simulink model "psb2machinesSVC_PSS"  (Simulink 6.0)
settings: Solver=ode23tb  StartTime=0.0  StopTime=10  MaxStep=1/60  RelTol=1e-3
InitFcn:
  | powericon('psbinitsys',bdroot);
undefined symbols (not defined in the file or in its folder): D1, Delta, gcbh, powericon
libraries: powerlib2 x23, powerlib_extras x5
settings Model: Creator=sybille  LastModifiedBy=batserve  ExtModeTrigMode=oneshot  ExtModeArmWhenConnect=off  ExtModeAutoUpdateStatusClock=off
settings DataIOCC: LimitDataPoints=off  SignalLoggingName=sigsOut
settings OptimizationCC: BlockReduction=off  BooleanDataType=off
settings DebuggingCC: SolverPrmCheckMsg=none
settings HardwareCC: TargetUnknown=on

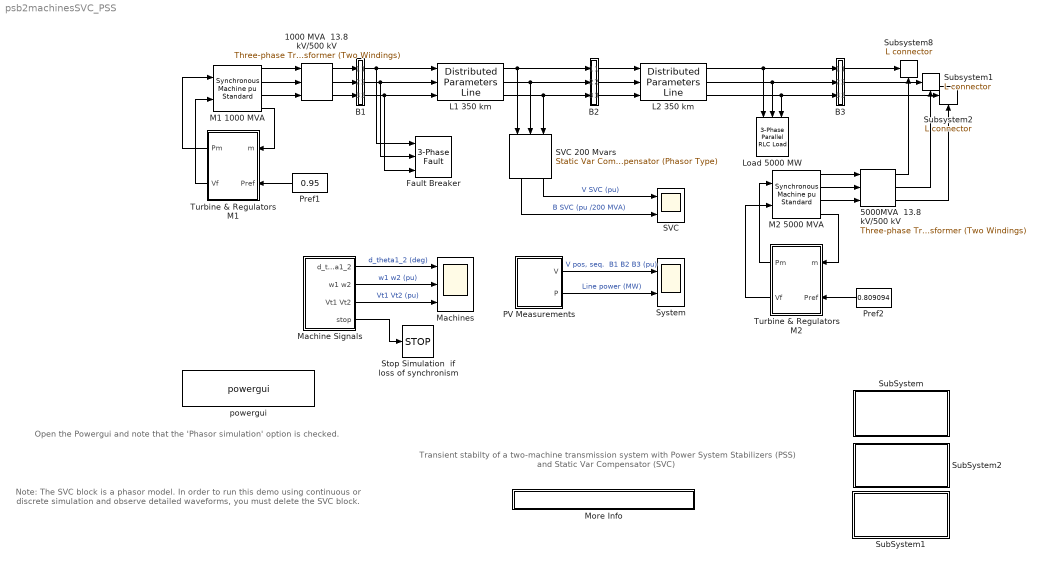
== system psb2machinesSVC_PSS ==
  note: Transient stabilty of a two-machine transmission system
      | with Power System Stabilizers (PSS)
      | and Static Var Compensator (SVC)
  note: Open the Powergui and note
      | that the 'Phasor simulation'
      | option is checked.
  note: Note:
      | The SVC block is a phasor model.
      | In order to run this demo using
      | continuous or discrete simulation
      | and observe detailed waveforms,
      | you must delete the SVC block.
  1000 MVA  13.8 kV/500 kV : powerlib2/Elements/Three-phase Transformer (Two Windings)  Tag=PoWeRsYsTeMbLoCk  nominal=[ 1000e6 60 ]  type1=Delta (D1)  params1="[ 13.8e3 0.002  0.0]"  type2=Yg  params2=[ 500e3 0.002 0.12]  ynsat=off  rmag=500  lm=500  sat="[ 0,0  ;  0.005,1.2  ;  1.0,1.4 ]"  hyst=off  matfile='hysteresis'  sif=off  phi0=[ 0.8 , -0.8 , 0.7 ]  initialslopes=[+1 +1 +1]  mesure=None  PSBOutputType=1111
  5000MVA  13.8 kV/500 kV : powerlib2/Elements/Three-phase Transformer (Two Windings)  Tag=PoWeRsYsTeMbLoCk  nominal=[ 5000e6 60 ]  type1=Delta (D1)  params1="[ 13.8e3 0.002  0.0]"  type2=Yg  params2=[ 500e3 0.002 0.12]  ynsat=off  rmag=500  lm=500  sat="[ 0,0  ;  0.005,1.2  ;  1.0,1.4 ]"  hyst=off  matfile='hysteresis'  sif=off  phi0=[ 0.8 , -0.8 , 0.7 ]  initialslopes=[+1 +1 +1]  mesure=None  PSBOutputType=1111
  B1 : Subsystem  Tag=PoWeRsYsTeMmEaSuReMeNt  AncestorBlock=powerlib2/Measurements/Three-Phase V-I Measurement  LoadFcn=powericon('psbloadfunction',gcbh,'3-Phase VI Measurement','');  InitFcn=powericon('checksum',bdroot)  mask(3-Phase VI Measurement){VChoice=phase-to-ground, ualv=on, labelV=Vabc_B1, Vpu=on, Vbase=500e3, IChoice=yes, ualc=on, labelC=Iabc_B1, Ppu=on, Pbase=100e6, OutputType=Complex, PhasorSimulation=on, PSBequivalent=0, PSBOutputType=11100}
      mask prompts: VChoice "Voltage measurement"; ualv "Use a label"; labelV "Signal label  (use a From block to collect signal)"; Vpu "Voltage  in pu"; Vbase "Base voltage (Vrms phase-phase) :"; IChoice "Current measurement"; ualc "Use a label"; labelC "Signal label  (use a From block to collect signal)"; Ppu "Currents in pu"; Pbase "Base power ( VA 3 phase)"; OutputType "Output signal :"; PhasorSimulation "Phasor simulation"; PSBequivalent "Equivalent circuit"
      mask help:
      | This block is used to measure three-phase voltages and currents in a circuit. When connected in series with a three-phase element, it return the three phase-to-ground voltages and line currents.
      |
      | The block can output the voltages and currents in per unit values or in volts and amperes. Check the appropriate boxes if you want to output the voltages and currents  in pu
      mask init:
      | powericon('psbcallbacks',gcb,'Three-phase measurements',4);
      | if  Vpu
      |     xKv=1/(Vbase/sqrt(3)*sqrt(2));
      | else
      |     xKv=1;
      | end
      | if  Ppu
      |     xKi=1/(Pbase/Vbase/sqrt(3)*sqrt(2));
      | else
      |     xKi=1;
      | end
      | switch OutputType
      | case 1
      |     OutputSelection  = [1:6];
      |     PhasorModeV = [1:3];
      |     NormalModeV = [7:9];
      |     PhasorModeI = [4:6];
      |     NormalModeI = [10:12];
      |     Kv = xKv;
      |     Ki = xKi;
      | case 2
      |     OutputSelection = [7,13,8,14,9,15,10,16,11,17,12,18];
      |     PhasorModeV = [1:6];
      |     NormalModeV = [13:15];
      |     PhasorModeI = [7:12];
      |     NormalModeI = [16:18];
      |     Kv = xKv;
      |     Ki = xKi;
      | case 3
      |     OutputSelection = [13,19,14,20,15,21,16,22,17,23,18,24];
      |     PhasorModeV = [1:6];
      |     NormalModeV = [13:15];
      |     PhasorModeI = [7:12];
      |     NormalModeI = [16:18];
      |     Kv = [xKv 1 xKv 1 xKv 1];
      |     Ki = [xKi 1 xKi 1 xKi 1];
      | case 4
      |     OutputSelection  = [19:24];
      |     PhasorModeV = [1:3];
      |     NormalModeV = [7:9];
      |     PhasorModeI = [4:6];
      |     NormalModeI = [10:12];
      |     Kv = xKv;
      |     Ki = xKi;
      | end
      | if PhasorSimulation
      |     SelectionModeV = PhasorModeV;
      |     SelectionModeI = PhasorModeI;
      | else
      |     SelectionModeV = NormalModeV;
      |     SelectionModeI = NormalModeI;
      |     Kv = xKv;
      |     Ki = xKi;
      | end
      settings: CopyFcn=powericon('psbloadfunction',gcbh,'3-Phase VI Measurement','VerifyPhasor');  CloseFcn=%3phaseVImeasurement
      mask Help: web(psbhelp)
      mask StyleString: popup(no|phase-to-ground|phase-to-phase),checkbox,edit,checkbox,edit,popup(no|yes),checkbox,edit,checkbox,edit,popup(Complex|Real-Imag|Magnitude-Angle|Magnitude),checkbox,edit,edit
      mask CallbackString: powericon('psbcallbacks',gcb,'Three-phase measurements',2);|powericon('psbcallbacks',gcb,'Three-phase measurements',2);||powericon('psbcallbacks',gcb,'Three-phase measurements',2);||powericon('psbcallbacks',gcb,'Three-phase measurements',2);|powericon('psbcallbacks',gcb,'Three-phase measurements',2);||powericon('psbcallbacks',gcb,'Three-phase measurements',4);|||||
  B2 : Subsystem  Tag=PoWeRsYsTeMmEaSuReMeNt  AncestorBlock=powerlib2/Measurements/Three-Phase V-I Measurement  LoadFcn=powericon('psbloadfunction',gcbh,'3-Phase VI Measurement','');  InitFcn=powericon('checksum',bdroot)  mask(3-Phase VI Measurement){VChoice=phase-to-ground, ualv=on, labelV=Vabc_B2, Vpu=on, Vbase=500e3, IChoice=no, ualc=off, labelC=I1, Ppu=off, Pbase=100e6, OutputType=Complex, PhasorSimulation=on, PSBequivalent=0, PSBOutputType=11100}
      mask prompts: VChoice "Voltage measurement"; ualv "Use a label"; labelV "Signal label  (use a From block to collect signal)"; Vpu "Voltage  in pu"; Vbase "Base voltage (Vrms phase-phase) :"; IChoice "Current measurement"; ualc "Use a label"; labelC "Signal label  (use a From block to collect signal)"; Ppu "Currents in pu"; Pbase "Base power ( VA 3 phase)"; OutputType "Output signal :"; PhasorSimulation "Phasor simulation"; PSBequivalent "Equivalent circuit"
      mask help:
      | This block is used to measure three-phase voltages and currents in a circuit. When connected in series with a three-phase element, it return the three phase-to-ground voltages and line currents.
      |
      | The block can output the voltages and currents in per unit values or in volts and amperes. Check the appropriate boxes if you want to output the voltages and currents  in pu
      mask init: same as psb2machinesSVC_PSS/B1
      settings: CopyFcn=powericon('psbloadfunction',gcbh,'3-Phase VI Measurement','VerifyPhasor');  CloseFcn=%3phaseVImeasurement
      mask Help: web(psbhelp)
      mask StyleString: popup(no|phase-to-ground|phase-to-phase),checkbox,edit,checkbox,edit,popup(no|yes),checkbox,edit,checkbox,edit,popup(Complex|Real-Imag|Magnitude-Angle|Magnitude),checkbox,edit,edit
      mask CallbackString: powericon('psbcallbacks',gcb,'Three-phase measurements',2);|powericon('psbcallbacks',gcb,'Three-phase measurements',2);||powericon('psbcallbacks',gcb,'Three-phase measurements',2);||powericon('psbcallbacks',gcb,'Three-phase measurements',2);|powericon('psbcallbacks',gcb,'Three-phase measurements',2);||powericon('psbcallbacks',gcb,'Three-phase measurements',4);|||||
  B3 : Subsystem  Tag=PoWeRsYsTeMmEaSuReMeNt  AncestorBlock=powerlib2/Measurements/Three-Phase V-I Measurement  LoadFcn=powericon('psbloadfunction',gcbh,'3-Phase VI Measurement','');  InitFcn=powericon('checksum',bdroot)  mask(3-Phase VI Measurement){VChoice=phase-to-ground, ualv=on, labelV=Vabc_B3, Vpu=on, Vbase=500e3, IChoice=no, ualc=off, labelC=I1, Ppu=off, Pbase=100e6, OutputType=Complex, PhasorSimulation=on, PSBequivalent=0, PSBOutputType=11100}
      mask prompts: VChoice "Voltage measurement"; ualv "Use a label"; labelV "Signal label  (use a From block to collect signal)"; Vpu "Voltage  in pu"; Vbase "Base voltage (Vrms phase-phase) :"; IChoice "Current measurement"; ualc "Use a label"; labelC "Signal label  (use a From block to collect signal)"; Ppu "Currents in pu"; Pbase "Base power ( VA 3 phase)"; OutputType "Output signal :"; PhasorSimulation "Phasor simulation"; PSBequivalent "Equivalent circuit"
      mask help:
      | This block is used to measure three-phase voltages and currents in a circuit. When connected in series with a three-phase element, it return the three phase-to-ground voltages and line currents.
      |
      | The block can output the voltages and currents in per unit values or in volts and amperes. Check the appropriate boxes if you want to output the voltages and currents  in pu
      mask init: same as psb2machinesSVC_PSS/B1
      settings: CopyFcn=powericon('psbloadfunction',gcbh,'3-Phase VI Measurement','VerifyPhasor');  CloseFcn=%3phaseVImeasurement
      mask Help: web(psbhelp)
      mask StyleString: popup(no|phase-to-ground|phase-to-phase),checkbox,edit,checkbox,edit,popup(no|yes),checkbox,edit,checkbox,edit,popup(Complex|Real-Imag|Magnitude-Angle|Magnitude),checkbox,edit,edit
      mask CallbackString: powericon('psbcallbacks',gcb,'Three-phase measurements',2);|powericon('psbcallbacks',gcb,'Three-phase measurements',2);||powericon('psbcallbacks',gcb,'Three-phase measurements',2);||powericon('psbcallbacks',gcb,'Three-phase measurements',2);|powericon('psbcallbacks',gcb,'Three-phase measurements',2);||powericon('psbcallbacks',gcb,'Three-phase measurements',4);|||||
  Fault Breaker : powerlib2/Elements/3-Phase Fault  sa=on  sb=off  sc=off  Rdef=0.001  st=on  Rt=0.001  comext=off  sw_status=[1 0]  sw_times=[ 0.1 0.1+6.0/60]  Ts=0  init_statext=[0 0 1]  Rp=1e6  Cp=inf  mesure=None
  L1 350 km : powerlib2/Elements/Distributed Parameters Line  Tag=PoWeRsYsTeMbLoCk  n=3  f=60  r="[0.01755  0.2758]"  l="[0.8737e-3  3.220e-3]"  c="[13.33e-9  8.297e-9]"  lgt=350  x1=[0 -1.745e-008 4.874e+005 -1.124e+005;0.0003618 -1.101e-008 4.982e+005 -4.51e+004;0.0007236 -4.365e-009 4.997e+005 2.307e+004;0.001085 2.363e-009 4.919e+005 9.08e+004;0.001447 9.047e-009 4.75e+005 1.569e+005;0.001809 1.556e-008 4.493e+005 2.2e+005]  x2=[0 8.099e-009 4.009e+005 -3.067e+005;0.0003618 7.338e-009 4.389e+005 -2.493e+005;0.0007236 6.44e-009 4.687e+005 -1.873e+005;0.001085 5.423e-009 4.898e+005 -1.218e+005;0.001447 4.305e-009 5.019e+005 -5.41e+004;0.001809 3.107e-009 5.046e+005 1.464e+004]  x3=[0 7.745e-011 13.12 -184.5;0.0003618 8.905e-011 38.08 -181;0.0007236 9.899e-011 62.33 -174.1;0.001085 1.071e-010 85.43 -164;0.001447 1.132e-010 106.9 -150.9;0.001809 1.172e-010 126.5 -134.9]  x4=[0 -1.132e-010 3024 -2208;0.0003618 -1.172e-010 3296 -1776;0.0007236 -1.19e-010 3507 -1312;0.001085 -1.186e-010 3652 -822.8;0.001447 -1.16e-010 3730 -318.5;0.001809 -1.113e-010 3739 191.7]  x5=0.001809  mesure=None  PSBOutputType=111111111111111111111111111111
  L2 350 km : powerlib2/Elements/Distributed Parameters Line  Tag=PoWeRsYsTeMbLoCk  n=3  f=60  r="[0.01755  0.2758]"  l="[0.8737e-3  3.220e-3]"  c="[13.33e-9  8.297e-9]"  lgt=350  x1=[0 8.099e-009 4.009e+005 -3.067e+005;0.0003618 7.338e-009 4.389e+005 -2.493e+005;0.0007236 6.44e-009 4.687e+005 -1.873e+005;0.001085 5.423e-009 4.898e+005 -1.218e+005;0.001447 4.305e-009 5.019e+005 -5.41e+004;0.001809 3.107e-009 5.046e+005 1.464e+004]  x2=[0 2.948e-008 2.377e+005 -4.356e+005;0.0003618 2.166e-008 2.947e+005 -3.992e+005;0.0007236 1.345e-008 3.463e+005 -3.555e+005;0.001085 4.977e-009 3.914e+005 -3.051e+005;0.001447 -3.584e-009 4.292e+005 -2.49e+005;0.001809 -1.208e-008 4.591e+005 -1.883e+005]  x3=[0 1.376e-010 52.72 -145;0.0003618 1.394e-010 71.94 -136.5;0.0007236 1.386e-010 89.83 -125.4;0.001085 1.352e-010 106.1 -112;0.001447 1.292e-010 120.3 -96.59;0.001809 1.209e-010 132.3 -79.33]  x4=[0 -5.233e-011 1740 -3266;0.0003618 -6.396e-011 2168 -2999;0.0007236 -7.44e-011 2556 -2677;0.001085 -8.346e-011 2896 -2304;0.001447 -9.097e-011 3183 -1889;0.001809 -9.679e-011 3410 -1439]  x5=0.001809  mesure=None  PSBOutputType=111111111111111111111111111111
  Load 5000 MW : powerlib2/Elements/3-Phase Parallel RLC Load  Orientation=down  Vpp=500e3  fn=60  P3=5000e6  QL3=0  QC3=0
  M1 1000 MVA : powerlib2/Machines/Synchronous Machine pu Standard  Tag=PoWeRsYsTeMbLoCk  rotorType=Salient-pole  x1="[1000E6  13800   60 ]"  x2b=[ 31 32 33 34 35 36 37 ]  x2=[ 1.305, 0.296, 0.252, 0.474, 0.243, 0.18 ]  dAxisT=Short-circuit  qAxisT=Open-circuit  x3a=[]  x3b=[]  x3c=[]  x3d=[]  x3=[ 1.01, 0.053, 0.1 ]  x3e=[]  x3f=[]  x3g=[]  x4=2.8544e-3  x5="[ 3.7 0  32]"  x6=[0 -16.6861 0.950218 0.950218 0.950218 48.1093 -71.8907 168.109 1.44424]  x7=off  x8=[0.6404,0.7127,0.8441,0.9214,0.9956,1.082,1.19,1.316,1.457;0.7,0.7698,0.8872,0.9466,0.9969,1.046,1.1,1.151,1.201]  PSBOutputType=1110  iounits=0.5  LoadFlowParameters=[1 950000000 0 0]
  M2 5000 MVA : powerlib2/Machines/Synchronous Machine pu Standard  Tag=PoWeRsYsTeMbLoCk  rotorType=Salient-pole  x1="[5000E6  13800   60 ]"  x2b=[ 31 32 33 34 35 36 37 ]  x2=[ 1.305, 0.296, 0.252, 0.474, 0.243, 0.18 ]  dAxisT=Short-circuit  qAxisT=Open-circuit  x3a=[]  x3b=[]  x3c=[]  x3d=[]  x3=[ 1.01, 0.053, 0.1 ]  x3e=[]  x3f=[]  x3g=[]  x4=2.8544e-3  x5="[ 3.7 0  32]"  x6=[0 -69.7487 0.812764 0.812764 0.812764 -5.44703 -125.447 114.553 1.40021]  x7=off  x8=[0.6404,0.7127,0.8441,0.9214,0.9956,1.082,1.19,1.316,1.457;0.7,0.7698,0.8872,0.9466,0.9969,1.046,1.1,1.151,1.201]  PSBOutputType=1110  iounits=0.5  LoadFlowParameters=[2 4000000000 0 0]
  Machine Signals : Subsystem
  Machines : Scope  NumInputPorts=3
      settings: TimeRange=10  YMin=30~0.995~0  YMax=70~1.005~1.4  SaveName=mach
  More Info : Subsystem
      settings: OpenFcn=Powerlib3root = which('psb2machinesSVC_PSS');PSBroot = Powerlib3root(1:end-23);web([PSBroot,'psb2machines.html'])
      mask Display: disp('? : Double click here for more info')
  PV Measurements : Subsystem
  "Pref1 " : Constant  Orientation=left  Value=0.95
  Pref2 : Constant  Orientation=left  Value=0.809094
  SVC : Scope  NumInputPorts=2
      settings: TimeRange=10  YMin=0.7~-1  YMax=1.1~1  SaveName=svc
  SVC 200 Mvars : powerlib_extras/Phasor Library/Static Var Compensator (Phasor Type)  Orientation=down  mode=Fixed Susceptance  Vnom=500e3  Qnom=200e6  Bref=0.0  Vref=1.009  Xs=0.03  To=0.1  Tm=8e-3  Td=4e-3
  Stop Simulation  if loss of synchronism : Stop
  SubSystem : Subsystem
      settings: OpenFcn=openfig('psb2macSVC_PhasorVsDet.fig');
      mask Display: disp('Show comparison\nDetailed vs Phasor\n simulation')
  SubSystem1 : Subsystem
      settings: OpenFcn=openfig('psb2macSVC_3phfault.fig');
      mask Display: disp('Show impact of SVC\nfor 3-phase fault')
  SubSystem2 : Subsystem
      settings: OpenFcn=openfig('psb2macSVC_1phfault.fig');
      mask Display: disp('Show impact of PSS\nfor 1-phase fault')
  Subsystem1 : powerlib2/Connectors/L connector  Tag=PoWeRsYsTeMbLoCk  Orientation=up
  Subsystem2 : powerlib2/Connectors/L connector  Tag=PoWeRsYsTeMbLoCk  Orientation=up
  Subsystem8 : powerlib2/Connectors/L connector  Tag=PoWeRsYsTeMbLoCk  Orientation=up
  System : Scope  NumInputPorts=2
      settings: TimeRange=10  YMin=0~0  YMax=1.5~1500  SaveName=mach1
  Turbine & Regulators M1 : Subsystem  Orientation=left
  Turbine & Regulators M2 : Subsystem  Orientation=left
  powergui : powerlib2/powergui  Frange=[0:2:500]  Ylog=off  Xlog=off  save=off  variable=ZData  ZoomFFT=on  StartTime=0.0  cycles=1  DisplayStyle=off  fundamental=60  FreqAxis=off  MaxFrequency=1000  frequencyindice=1  frequencyindicesteady=1  RmsSteady=1  display=off  Ts=0  methode=on  frequency=60  echomessages=off
  wires:
  M1 1000 MVA/1 -> 1000 MVA  13.8 kV/500 kV/1
  M1 1000 MVA/2 -> 1000 MVA  13.8 kV/500 kV/2
  M1 1000 MVA/3 -> 1000 MVA  13.8 kV/500 kV/3
  M1 1000 MVA/4 -> Turbine & Regulators M1/1(m)
  Turbine & Regulators M1/1(Pm) -> M1 1000 MVA/1
  Turbine & Regulators M1/2(Vf) -> M1 1000 MVA/2
  5000MVA  13.8 kV/500 kV/1 -> Subsystem8/1
  5000MVA  13.8 kV/500 kV/2 -> Subsystem1/1
  5000MVA  13.8 kV/500 kV/3 -> Subsystem2/1
  M2 5000 MVA/1 -> 5000MVA  13.8 kV/500 kV/1
  M2 5000 MVA/2 -> 5000MVA  13.8 kV/500 kV/2
  M2 5000 MVA/3 -> 5000MVA  13.8 kV/500 kV/3
  SVC 200 Mvars/2 -> SVC/1  "V SVC (pu)"
  SVC 200 Mvars/1 -> SVC/2  "B SVC (pu /200 MVA)"
  L2 350 km/1 -> B3/1(A), Load 5000 MW/1
  L2 350 km/2 -> B3/2(B), Load 5000 MW/2
  L2 350 km/3 -> B3/3(C), Load 5000 MW/3
  1000 MVA  13.8 kV/500 kV/1 -> B1/1(A)
  1000 MVA  13.8 kV/500 kV/2 -> B1/2(B)
  1000 MVA  13.8 kV/500 kV/3 -> B1/3(C)
  L1 350 km/2 -> B2/2(B), SVC 200 Mvars/2
  L1 350 km/1 -> B2/1(A), SVC 200 Mvars/1
  L1 350 km/3 -> B2/3(C), SVC 200 Mvars/3
  Turbine & Regulators M2/1(Pm) -> M2 5000 MVA/1
  Turbine & Regulators M2/2(Vf) -> M2 5000 MVA/2
  M2 5000 MVA/4 -> Turbine & Regulators M2/1(m)
  Pref2/1 -> Turbine & Regulators M2/2(Pref)
  Machine Signals/2(w1 w2) -> Machines/2  "w1 w2 (pu)"
  Machine Signals/1(d_theta1_2) -> Machines/1  "d_theta1_2 (deg)"
  Machine Signals/4(stop) -> Stop Simulation  if loss of synchronism/1
  Machine Signals/3(Vt1 Vt2) -> Machines/3  "Vt1 Vt2 (pu)"
  "Pref1 "/1 -> Turbine & Regulators M1/2(Pref)
  B2/1("A ") -> L2 350 km/1
  B2/2("B ") -> L2 350 km/2
  B2/3("C ") -> L2 350 km/3
  B1/1("A ") -> Fault Breaker/1, L1 350 km/1
  B1/2("B ") -> Fault Breaker/2, L1 350 km/2
  B1/3("C ") -> Fault Breaker/3, L1 350 km/3
  B3/1("A ") -> Subsystem8/Enable
  B3/2("B ") -> Subsystem1/Enable
  B3/3("C ") -> Subsystem2/Enable
  PV Measurements/1(V) -> System/1  "V pos, seq.  B1 B2 B3 (pu)"
  PV Measurements/2(P) -> System/2  "Line power (MW)"

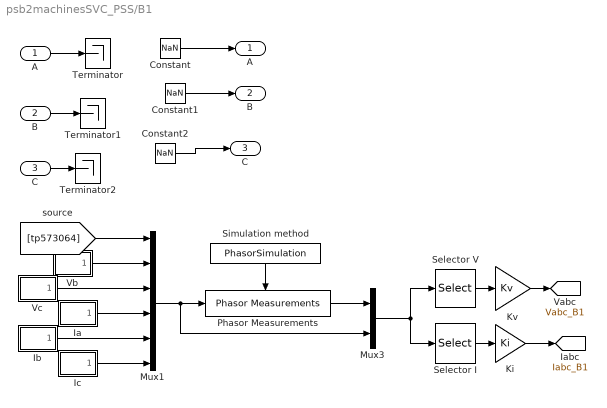
== system psb2machinesSVC_PSS/B1 ==
  A : Inport  Port=1  LatchInput=off
  B : Inport  Port=2  LatchInput=off
  C : Inport  Port=3  LatchInput=off
  Constant : Constant  Value=NaN
  Constant1 : Constant  Value=NaN
  Constant2 : Constant  Value=NaN
  Ia : Subsystem  AncestorBlock=powerlib2/Measurements/Three-Phase V-I Measurement/Ia
  Ib : Subsystem  AncestorBlock=powerlib2/Measurements/Three-Phase V-I Measurement/Ib
  Ic : Subsystem  AncestorBlock=powerlib2/Measurements/Three-Phase V-I Measurement/Ic
  Ki : Gain  Gain=Ki  SaturateOnIntegerOverflow=on
  Kv : Gain  Gain=Kv  SaturateOnIntegerOverflow=on
  Mux1 : Mux  Inputs=6
  Mux3 : Mux  Inputs=2
  Phasor Measurements : powerlib2/Measurements/Three-Phase V-I Measurement/Phasor Measurements  TreatAsAtomicUnit=on  SimViewingDevice=off  DataTypeOverride=UseLocalSettings  MinMaxOverflowLogging=UseLocalSettings
      settings: Permissions=ReadWrite  RTWFcnNameOpts=Auto  RTWFileNameOpts=Auto
  Selector I : Selector  Elements=SelectionModeI  InputPortWidth=length(OutputSelection)+6
  Selector V : Selector  Elements=SelectionModeV  InputPortWidth=length(OutputSelection)+6
  Simulation method : Constant  Orientation=down  Value=PhasorSimulation
  Terminator : Terminator
  Terminator1 : Terminator
  Terminator2 : Terminator
  Vb : Subsystem  AncestorBlock=powerlib2/Measurements/Three-Phase V-I Measurement/Vb
  Vc : Subsystem  AncestorBlock=powerlib2/Measurements/Three-Phase V-I Measurement/Vc
  "A " : Outport
  "B " : Outport  Port=2
  "C " : Outport  Port=3
  tag scope: Iabc_B1=global, Vabc_B1=global
  wires:
  A/1 -> Terminator/1
  B/1 -> Terminator1/1
  C/1 -> Terminator2/1
  Constant/1 -> "A "/1
  Constant1/1 -> "B "/1
  Constant2/1 -> "C "/1
  Kv/1 -> [Vabc_B1]
  Ki/1 -> [Iabc_B1]
  Selector V/1 -> Kv/1
  Selector I/1 -> Ki/1
  Mux3/1 -> Selector I/1, Selector V/1
  Phasor Measurements/1 -> Mux3/1
  Simulation method/1 -> Phasor Measurements/Enable
  Mux1/1 -> Mux3/2, Phasor Measurements/1
  [tp573064] -> Mux1/1
  Vb/1(Out1) -> Mux1/2
  Vc/1(Out1) -> Mux1/3
  Ia/1(Out1) -> Mux1/4
  Ib/1(Out1) -> Mux1/5
  Ic/1(Out1) -> Mux1/6

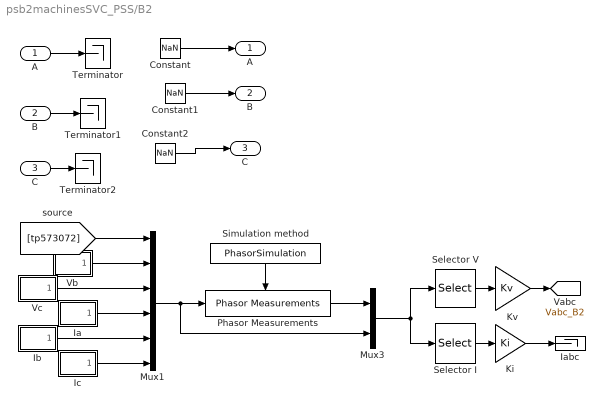
== system psb2machinesSVC_PSS/B2 ==
  A : Inport  Port=1  LatchInput=off
  B : Inport  Port=2  LatchInput=off
  C : Inport  Port=3  LatchInput=off
  Constant : Constant  Value=NaN
  Constant1 : Constant  Value=NaN
  Constant2 : Constant  Value=NaN
  Ia : Subsystem  AncestorBlock=powerlib2/Measurements/Three-Phase V-I Measurement/Ia
  Iabc : Terminator
  Ib : Subsystem  AncestorBlock=powerlib2/Measurements/Three-Phase V-I Measurement/Ib
  Ic : Subsystem  AncestorBlock=powerlib2/Measurements/Three-Phase V-I Measurement/Ic
  Ki : Gain  Gain=Ki  SaturateOnIntegerOverflow=on
  Kv : Gain  Gain=Kv  SaturateOnIntegerOverflow=on
  Mux1 : Mux  Inputs=6
  Mux3 : Mux  Inputs=2
  Phasor Measurements : powerlib2/Measurements/Three-Phase V-I Measurement/Phasor Measurements  TreatAsAtomicUnit=on  SimViewingDevice=off  DataTypeOverride=UseLocalSettings  MinMaxOverflowLogging=UseLocalSettings
      settings: Permissions=ReadWrite  RTWFcnNameOpts=Auto  RTWFileNameOpts=Auto
  Selector I : Selector  Elements=SelectionModeI  InputPortWidth=length(OutputSelection)+6
  Selector V : Selector  Elements=SelectionModeV  InputPortWidth=length(OutputSelection)+6
  Simulation method : Constant  Orientation=down  Value=PhasorSimulation
  Terminator : Terminator
  Terminator1 : Terminator
  Terminator2 : Terminator
  Vb : Subsystem  AncestorBlock=powerlib2/Measurements/Three-Phase V-I Measurement/Vb
  Vc : Subsystem  AncestorBlock=powerlib2/Measurements/Three-Phase V-I Measurement/Vc
  "A " : Outport
  "B " : Outport  Port=2
  "C " : Outport  Port=3
  tag scope: Vabc_B2=global
  wires:
  Ic/1(Out1) -> Mux1/6
  Ib/1(Out1) -> Mux1/5
  Ia/1(Out1) -> Mux1/4
  Vc/1(Out1) -> Mux1/3
  Vb/1(Out1) -> Mux1/2
  [tp573072] -> Mux1/1
  Mux1/1 -> Phasor Measurements/1, Mux3/2
  Simulation method/1 -> Phasor Measurements/Enable
  Phasor Measurements/1 -> Mux3/1
  Mux3/1 -> Selector V/1, Selector I/1
  Selector I/1 -> Ki/1
  Selector V/1 -> Kv/1
  Ki/1 -> Iabc/1
  Kv/1 -> [Vabc_B2]
  Constant2/1 -> "C "/1
  Constant1/1 -> "B "/1
  Constant/1 -> "A "/1
  C/1 -> Terminator2/1
  B/1 -> Terminator1/1
  A/1 -> Terminator/1

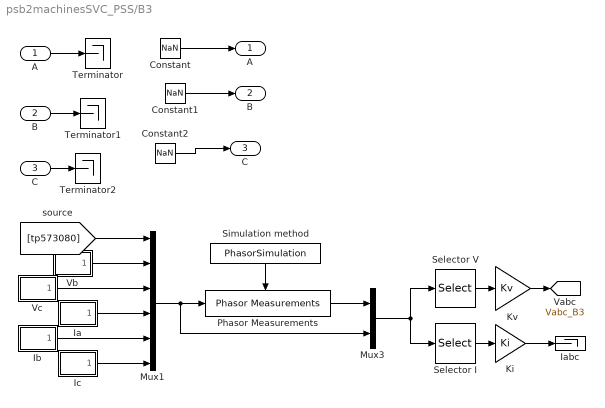
== system psb2machinesSVC_PSS/B3 ==
  A : Inport  Port=1  LatchInput=off
  B : Inport  Port=2  LatchInput=off
  C : Inport  Port=3  LatchInput=off
  Constant : Constant  Value=NaN
  Constant1 : Constant  Value=NaN
  Constant2 : Constant  Value=NaN
  Ia : Subsystem  AncestorBlock=powerlib2/Measurements/Three-Phase V-I Measurement/Ia
  Iabc : Terminator
  Ib : Subsystem  AncestorBlock=powerlib2/Measurements/Three-Phase V-I Measurement/Ib
  Ic : Subsystem  AncestorBlock=powerlib2/Measurements/Three-Phase V-I Measurement/Ic
  Ki : Gain  Gain=Ki  SaturateOnIntegerOverflow=on
  Kv : Gain  Gain=Kv  SaturateOnIntegerOverflow=on
  Mux1 : Mux  Inputs=6
  Mux3 : Mux  Inputs=2
  Phasor Measurements : powerlib2/Measurements/Three-Phase V-I Measurement/Phasor Measurements  TreatAsAtomicUnit=on  SimViewingDevice=off  DataTypeOverride=UseLocalSettings  MinMaxOverflowLogging=UseLocalSettings
      settings: Permissions=ReadWrite  RTWFcnNameOpts=Auto  RTWFileNameOpts=Auto
  Selector I : Selector  Elements=SelectionModeI  InputPortWidth=length(OutputSelection)+6
  Selector V : Selector  Elements=SelectionModeV  InputPortWidth=length(OutputSelection)+6
  Simulation method : Constant  Orientation=down  Value=PhasorSimulation
  Terminator : Terminator
  Terminator1 : Terminator
  Terminator2 : Terminator
  Vb : Subsystem  AncestorBlock=powerlib2/Measurements/Three-Phase V-I Measurement/Vb
  Vc : Subsystem  AncestorBlock=powerlib2/Measurements/Three-Phase V-I Measurement/Vc
  "A " : Outport
  "B " : Outport  Port=2
  "C " : Outport  Port=3
  tag scope: Vabc_B3=global
  wires:
  A/1 -> Terminator/1
  B/1 -> Terminator1/1
  C/1 -> Terminator2/1
  Constant/1 -> "A "/1
  Constant1/1 -> "B "/1
  Constant2/1 -> "C "/1
  Kv/1 -> [Vabc_B3]
  Ki/1 -> Iabc/1
  Selector V/1 -> Kv/1
  Selector I/1 -> Ki/1
  Mux3/1 -> Selector I/1, Selector V/1
  Phasor Measurements/1 -> Mux3/1
  Simulation method/1 -> Phasor Measurements/Enable
  Mux1/1 -> Mux3/2, Phasor Measurements/1
  [tp573080] -> Mux1/1
  Vb/1(Out1) -> Mux1/2
  Vc/1(Out1) -> Mux1/3
  Ia/1(Out1) -> Mux1/4
  Ib/1(Out1) -> Mux1/5
  Ic/1(Out1) -> Mux1/6

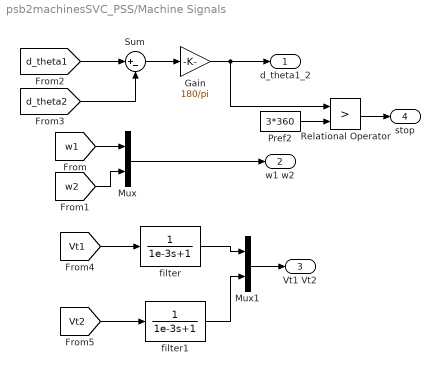
== system psb2machinesSVC_PSS/Machine Signals ==
  " filter" : TransferFcn  Denominator=[1e-3 1]
  " filter1" : TransferFcn  Denominator=[1e-3 1]
  Gain : Gain  Gain=180/pi  SaturateOnIntegerOverflow=on
  Mux : Mux  Inputs=2
  Mux1 : Mux  Inputs=2
  Pref2 : Constant  Value=3*360
  Relational Operator : RelationalOperator  Operator=>  InputSameDT=on
  Sum : Sum  Inputs=|+-  SaturateOnIntegerOverflow=on  InputSameDT=on
  d_theta1_2 : Outport
  w1 w2 : Outport  Port=2
  Vt1 Vt2 : Outport  Port=3
  stop : Outport  Port=4
  wires:
  " filter1"/1 -> Mux1/2
  " filter"/1 -> Mux1/1
  Relational Operator/1 -> stop/1
  Pref2/1 -> Relational Operator/2
  [Vt2] -> " filter1"/1
  Mux1/1 -> Vt1 Vt2/1
  [Vt1] -> " filter"/1
  [d_theta2] -> Sum/2
  [w2] -> Mux/2
  Gain/1 -> Relational Operator/1, d_theta1_2/1
  Mux/1 -> w1 w2/1
  [w1] -> Mux/1
  [d_theta1] -> Sum/1
  Sum/1 -> Gain/1

== system psb2machinesSVC_PSS/More Info ==

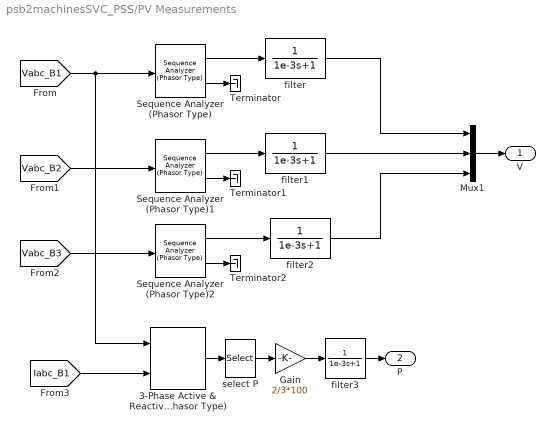
== system psb2machinesSVC_PSS/PV Measurements ==
   filter{,1..3} (4 alike) : TransferFcn  Denominator=[1e-3 1]
  3-Phase Active & Reactive Power (Phasor Type) : powerlib_extras/Phasor Library/3-Phase Active & Reactive Power (Phasor Type)
  Gain : Gain  Gain=2/3*100  SaturateOnIntegerOverflow=on
  Mux1 : Mux  Inputs=3
  Sequence Analyzer (Phasor Type) : powerlib_extras/Phasor Library/Sequence Analyzer (Phasor Type)  seq=Positive
  Sequence Analyzer (Phasor Type)1 : powerlib_extras/Phasor Library/Sequence Analyzer (Phasor Type)  seq=Positive
  Sequence Analyzer (Phasor Type)2 : powerlib_extras/Phasor Library/Sequence Analyzer (Phasor Type)  seq=Positive
  Terminator : Terminator
  Terminator1 : Terminator
  Terminator2 : Terminator
  select P : Selector  InputPortWidth=2
  V : Outport
  P : Outport  Port=2
  wires:
  " filter3"/1 -> P/1
  Gain/1 -> " filter3"/1
  3-Phase Active & Reactive Power (Phasor Type)/1 -> select P/1
  [Iabc_B1] -> 3-Phase Active & Reactive Power (Phasor Type)/2
  Sequence Analyzer (Phasor Type)2/2 -> Terminator2/1
  Sequence Analyzer (Phasor Type)1/2 -> Terminator1/1
  Sequence Analyzer (Phasor Type)/2 -> Terminator/1
  " filter2"/1 -> Mux1/3
  " filter1"/1 -> Mux1/2
  " filter"/1 -> Mux1/1
  Mux1/1 -> V/1
  Sequence Analyzer (Phasor Type)2/1 -> " filter2"/1
  Sequence Analyzer (Phasor Type)1/1 -> " filter1"/1
  [Vabc_B3] -> Sequence Analyzer (Phasor Type)2/1
  [Vabc_B2] -> Sequence Analyzer (Phasor Type)1/1
  Sequence Analyzer (Phasor Type)/1 -> " filter"/1
  [Vabc_B1] -> 3-Phase Active & Reactive Power (Phasor Type)/1, Sequence Analyzer (Phasor Type)/1
  select P/1 -> Gain/1

== system psb2machinesSVC_PSS/SubSystem ==

== system psb2machinesSVC_PSS/SubSystem1 ==

== system psb2machinesSVC_PSS/SubSystem2 ==

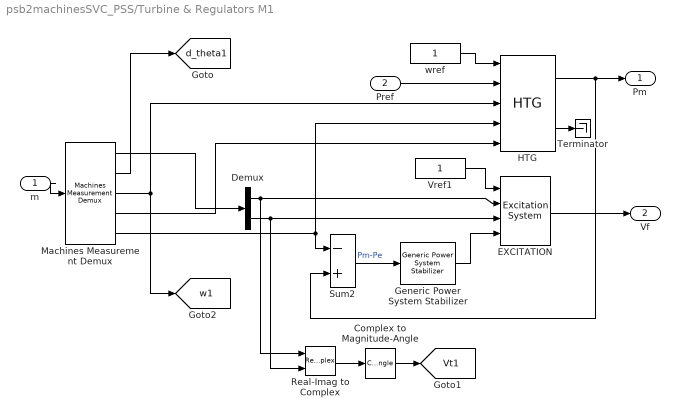
== system psb2machinesSVC_PSS/Turbine & Regulators M1 ==
  m : Inport  Port=1  LatchInput=off
  Pref : Inport  Port=2  LatchInput=off
  Complex to Magnitude-Angle : ComplexToMagnitudeAngle  Output=Magnitude
  Demux : Demux  Outputs=2
  EXCITATION : powerlib2/Machines/Excitation System  tr=20e-3  reg=[ 200, 0.001 ]  exc=[ 1, 0 ]  tgr=[ 0, 0 ]  damp=[ 0.001, 0.1 ]  sat=[ 0, 0 ]  lim="[ 0,  7, 0 ]"  v0=[1,1.44424]
  Generic Power System Stabilizer : powerlib2/Machines/Generic Power System Stabilizer  Tsensor=15e-3  K=2.5  Twashout=1  Tleadlag1=[60e-3 1]  Tleadlag2="[0  0]"  VSlimits=[-0.15 0.15]  Vinit=0  Plot_On=off  MagdB_On=on  FreqRange=logspace(-2,2,500)
  HTG : powerlib2/Machines/HTG  sm="[ 10/3  0.07 ]"  gate="[  0.01  0.97518  -0.1  0.1 ]"  reg="[  0.05  1.163  0.105  0  0.01  ]"  hyd="[  0  2.67  ]"  dref=0  po=0.952577
  Machines Measurement Demux : powerlib2/Machines/Machines Measurement Demux  machType=Synchronous  ssm1=on  ssm2=on  ssm3=on  ssm4=on  ssm5=on  ssm6=on  sm1=off  sm2=off  sm3=off  sm4=off  sm5=off  sm6=on  sm7=on  sm8=on  sm9=off  sm10=on  sm11=off  sm115=off  sm12=off  sm13=on  sm14=off  asm1=on  asm2=on  asm3=on  asm4=on  asm5=on  asm6=on  asm7=on  asm8=on  asm9=on  asm10=on  asm11=on  pmsm1=on  pmsm2=on  pmsm3=on  pmsm4=on  pmsm5=on  pmsm6=on  lastType=2
  Real-Imag to Complex : RealImagToComplex
  Sum2 : Sum  Inputs=-+  SaturateOnIntegerOverflow=on  InputSameDT=on
  Terminator : Terminator
  Vref1 : Constant
  wref : Constant
  Pm : Outport  InitialOutput=0
  Vf : Outport  Port=2  InitialOutput=0
  tag scope: Vt1=global, d_theta1=global, w1=global
  wires:
  Generic Power System Stabilizer/1 -> EXCITATION/4
  Machines Measurement Demux/5 -> Sum2/1, HTG/4
  Sum2/1 -> Generic Power System Stabilizer/1  "Pm-Pe"
  Machines Measurement Demux/2 -> [d_theta1]
  Complex to Magnitude-Angle/1 -> [Vt1]
  Demux/1 -> EXCITATION/2, Real-Imag to Complex/1
  EXCITATION/1 -> Vf/1
  Demux/2 -> EXCITATION/3, Real-Imag to Complex/2
  HTG/1 -> Sum2/2, Pm/1
  wref/1 -> HTG/1
  Pref/1 -> HTG/2
  Machines Measurement Demux/3 -> HTG/3, [w1]
  Machines Measurement Demux/4 -> HTG/5
  Machines Measurement Demux/1 -> Demux/1
  m/1 -> Machines Measurement Demux/1
  Vref1/1 -> EXCITATION/1
  HTG/2 -> Terminator/1
  Real-Imag to Complex/1 -> Complex to Magnitude-Angle/1

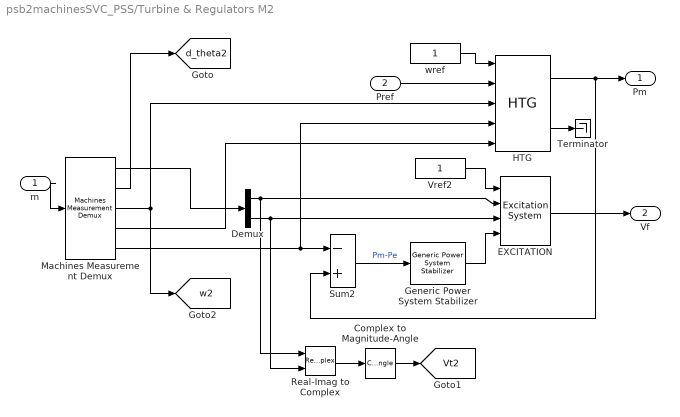
== system psb2machinesSVC_PSS/Turbine & Regulators M2 ==
  m : Inport  Port=1  LatchInput=off
  Pref : Inport  Port=2  LatchInput=off
  Complex to Magnitude-Angle : ComplexToMagnitudeAngle  Output=Magnitude
  Demux : Demux  Outputs=2
  EXCITATION : powerlib2/Machines/Excitation System  tr=20e-3  reg=[ 200, 0.001 ]  exc=[ 1, 0 ]  tgr=[ 0, 0 ]  damp=[ 0.001, 0.1 ]  sat=[ 0, 0 ]  lim="[ 0,  7, 0 ]"  v0=[1,1.40021]
  Generic Power System Stabilizer : powerlib2/Machines/Generic Power System Stabilizer  Tsensor=15e-3  K=2.5  Twashout=1  Tleadlag1=[60e-3 1]  Tleadlag2="[0  0]"  VSlimits=[-0.15 0.15]  Vinit=0  Plot_On=off  MagdB_On=on  FreqRange=logspace(-2,2,500)
  HTG : powerlib2/Machines/HTG  sm="[ 10/3  0.07 ]"  gate="[  0.01  0.97518  -0.1  0.1 ]"  reg="[  0.05  1.163  0.105  0  0.01  ]"  hyd="[  0  2.67  ]"  dref=0  po=0.810979
  Machines Measurement Demux : powerlib2/Machines/Machines Measurement Demux  machType=Synchronous  ssm1=on  ssm2=on  ssm3=on  ssm4=on  ssm5=on  ssm6=on  sm1=off  sm2=off  sm3=off  sm4=off  sm5=off  sm6=on  sm7=on  sm8=on  sm9=off  sm10=on  sm11=off  sm115=off  sm12=off  sm13=on  sm14=off  asm1=on  asm2=on  asm3=on  asm4=on  asm5=on  asm6=on  asm7=on  asm8=on  asm9=on  asm10=on  asm11=on  pmsm1=on  pmsm2=on  pmsm3=on  pmsm4=on  pmsm5=on  pmsm6=on  lastType=2
  Real-Imag to Complex : RealImagToComplex
  Sum2 : Sum  Inputs=-+  SaturateOnIntegerOverflow=on  InputSameDT=on
  Terminator : Terminator
  Vref2 : Constant
  wref : Constant
  Pm : Outport  InitialOutput=0
  Vf : Outport  Port=2  InitialOutput=0
  tag scope: Vt2=global, d_theta2=global, w2=global
  wires:
  Generic Power System Stabilizer/1 -> EXCITATION/4
  Real-Imag to Complex/1 -> Complex to Magnitude-Angle/1
  HTG/2 -> Terminator/1
  Vref2/1 -> EXCITATION/1
  m/1 -> Machines Measurement Demux/1
  Machines Measurement Demux/1 -> Demux/1
  Machines Measurement Demux/4 -> HTG/5
  Machines Measurement Demux/5 -> HTG/4, Sum2/1
  Machines Measurement Demux/3 -> [w2], HTG/3
  Pref/1 -> HTG/2
  wref/1 -> HTG/1
  HTG/1 -> Pm/1, Sum2/2
  Demux/2 -> Real-Imag to Complex/2, EXCITATION/3
  EXCITATION/1 -> Vf/1
  Demux/1 -> Real-Imag to Complex/1, EXCITATION/2
  Complex to Magnitude-Angle/1 -> [Vt2]
  Machines Measurement Demux/2 -> [d_theta2]
  Sum2/1 -> Generic Power System Stabilizer/1  "Pm-Pe"

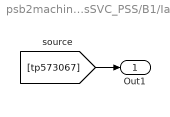
== system psb2machinesSVC_PSS/B1/Ia ==
  Out1 : Outport
  wires:
  [tp573067] -> Out1/1

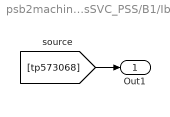
== system psb2machinesSVC_PSS/B1/Ib ==
  Out1 : Outport
  wires:
  [tp573068] -> Out1/1

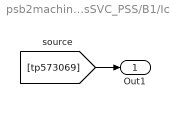
== system psb2machinesSVC_PSS/B1/Ic ==
  Out1 : Outport
  wires:
  [tp573069] -> Out1/1

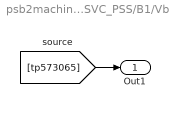
== system psb2machinesSVC_PSS/B1/Vb ==
  Out1 : Outport
  wires:
  [tp573065] -> Out1/1

== system psb2machinesSVC_PSS/B1/Vc ==
  Out1 : Outport
  wires:
  [tp573066] -> Out1/1

== system psb2machinesSVC_PSS/B2/Ia ==
  Out1 : Outport
  wires:
  [tp573075] -> Out1/1

== system psb2machinesSVC_PSS/B2/Ib ==
  Out1 : Outport
  wires:
  [tp573076] -> Out1/1

== system psb2machinesSVC_PSS/B2/Ic ==
  Out1 : Outport
  wires:
  [tp573077] -> Out1/1

== system psb2machinesSVC_PSS/B2/Vb ==
  Out1 : Outport
  wires:
  [tp573073] -> Out1/1

== system psb2machinesSVC_PSS/B2/Vc ==
  Out1 : Outport
  wires:
  [tp573074] -> Out1/1

== system psb2machinesSVC_PSS/B3/Ia ==
  Out1 : Outport
  wires:
  [tp573083] -> Out1/1

== system psb2machinesSVC_PSS/B3/Ib ==
  Out1 : Outport
  wires:
  [tp573084] -> Out1/1

== system psb2machinesSVC_PSS/B3/Ic ==
  Out1 : Outport
  wires:
  [tp573085] -> Out1/1

== system psb2machinesSVC_PSS/B3/Vb ==
  Out1 : Outport
  wires:
  [tp573081] -> Out1/1

== system psb2machinesSVC_PSS/B3/Vc ==
  Out1 : Outport
  wires:
  [tp573082] -> Out1/1
